simulink model "Sampling_switch_uncertainty"  (R2021b)
settings: Solver=VariableStepAuto  StartTime=0.0  StopTime=10.0  RelTol=1e-3
values from neighbouring files (symbols this model uses):
  bits_number = 13    [launch_pipeline_switch.m]
  cst = 2*pi*fin/1000    [launch_pipeline_switch.m]
  fin = antismear(fin_pre,fs,nfft)    [launch_pipeline_switch.m]
  ts = 1/fs    (= 1)    [launch_pipeline_switch.m]
(part 1 of 2)
settings Model: Creator=86151  LastModifiedBy=86151

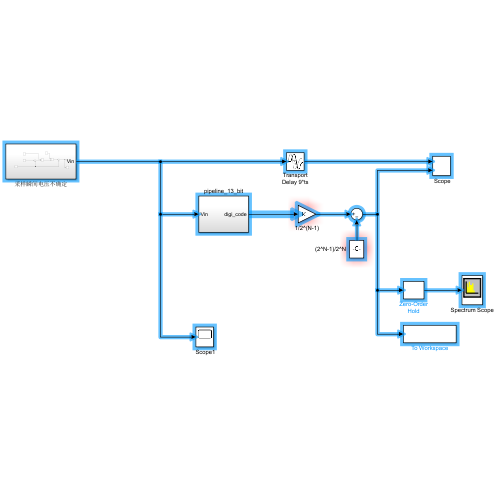
[thumbnail: Simulink's stored preview of the top-level diagram]
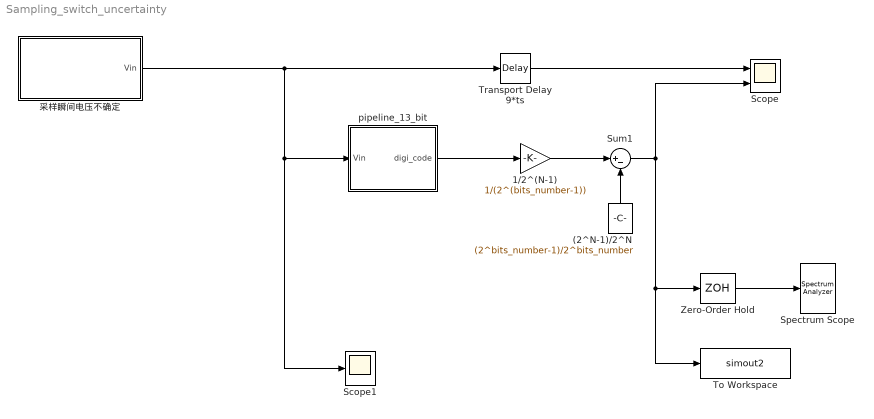
== system Sampling_switch_uncertainty ==
  " Scope" : Scope  NumInputPorts=2
  " Scope1" : Scope
  (2^N-1)/2^N : Constant  Value=(2^bits_number-1)/2^bits_number
  1/2^(N-1) : Gain  Gain=1/(2^(bits_number-1))
  Spectrum Scope : SpectrumAnalyzer
  Sum1 : Sum  Inputs=|+-
  To Workspace : ToWorkspace  VariableName=simout2  SampleTime=-1
  Transport Delay 9*ts : TransportDelay  DelayTime=9
  Zero-Order Hold : ZeroOrderHold
  pipeline_13_bit : Subsystem
  采样瞬间电压不确定 : Subsystem
  wires:
  采样瞬间电压不确定/1(Vin) -> " Scope1"/1, pipeline_13_bit/1(Vin), Transport Delay 9*ts/1
  Transport Delay 9*ts/1 -> " Scope"/1
  Zero-Order Hold/1 -> Spectrum Scope/1
  Sum1/1 -> " Scope"/2, To Workspace/1, Zero-Order Hold/1
  (2^N-1)/2^N/1 -> Sum1/2
  1/2^(N-1)/1 -> Sum1/1
  pipeline_13_bit/1(digi_code) -> 1/2^(N-1)/1

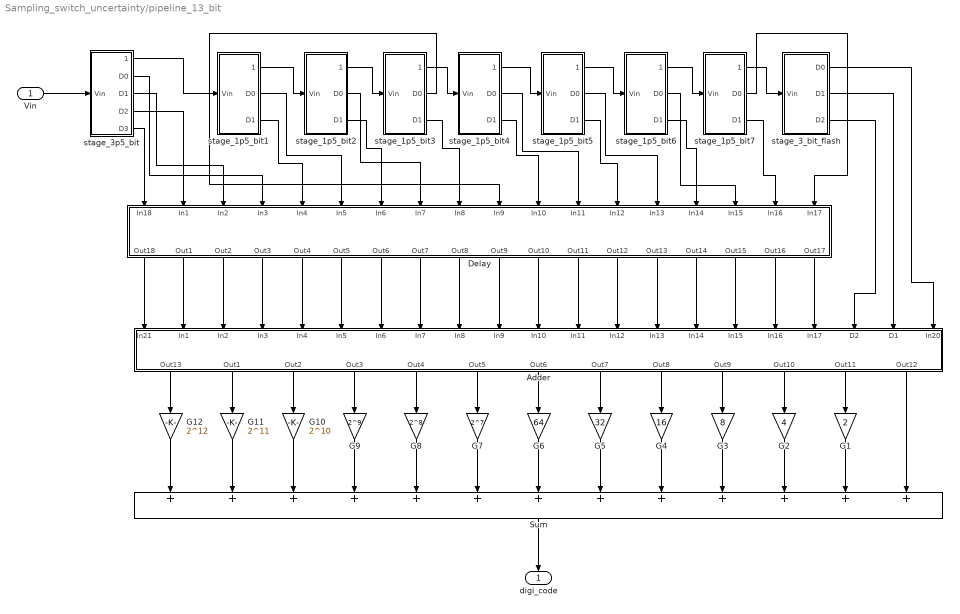
== system Sampling_switch_uncertainty/pipeline_13_bit ==
  Vin : Inport
  Adder : Subsystem
  Delay : Subsystem
  G1 : Gain  Gain=2
  G10 : Gain  Gain=2^10
  G11 : Gain  Gain=2^11
  G12 : Gain  Gain=2^12
  G2 : Gain  Gain=4
  G3 : Gain  Gain=8
  G4 : Gain  Gain=16
  G5 : Gain  Gain=32
  G6 : Gain  Gain=64
  G7 : Gain  Gain=2^7
  G8 : Gain  Gain=2^8
  G9 : Gain  Gain=2^9
  Sum : Sum  Inputs=+++++++++++++
  stage_1p5_bit1 : Subsystem
  stage_1p5_bit2 : Subsystem
  stage_1p5_bit3 : Subsystem
  stage_1p5_bit4 : Subsystem
  stage_1p5_bit5 : Subsystem
  stage_1p5_bit6 : Subsystem
  stage_1p5_bit7 : Subsystem
  stage_3_bit_flash : Subsystem
  stage_3p5_bit : Subsystem
  digi_code : Outport
  wires:
  G1/1 -> Sum/12
  stage_3p5_bit/4(D2) -> Delay/2(In1)
  stage_3p5_bit/3(D1) -> Delay/3(In2)
  stage_3p5_bit/2(D0) -> Delay/4(In3)
  stage_1p5_bit1/3(D1) -> Delay/5(In4)
  stage_1p5_bit1/2(D0) -> Delay/6(In5)
  stage_1p5_bit2/3(D1) -> Delay/7(In6)
  stage_1p5_bit2/2(D0) -> Delay/8(In7)
  G2/1 -> Sum/11
  G3/1 -> Sum/10
  G4/1 -> Sum/9
  G5/1 -> Sum/8
  G6/1 -> Sum/7
  G7/1 -> Sum/6
  G8/1 -> Sum/5
  G9/1 -> Sum/4
  G10/1 -> Sum/3
  G11/1 -> Sum/2
  stage_3_bit_flash/1(D0) -> Adder/21(In20)
  Adder/2(Out1) -> G11/1
  Adder/3(Out2) -> G10/1
  Adder/4(Out3) -> G9/1
  Adder/5(Out4) -> G8/1
  Adder/6(Out5) -> G7/1
  Adder/13(Out12) -> Sum/13
  Adder/12(Out11) -> G1/1
  Adder/11(Out10) -> G2/1
  Adder/10(Out9) -> G3/1
  Adder/9(Out8) -> G4/1
  Adder/8(Out7) -> G5/1
  Adder/7(Out6) -> G6/1
  stage_1p5_bit1/1(Residue) -> stage_1p5_bit2/1(Vin)
  stage_1p5_bit2/1(Residue) -> stage_1p5_bit3/1(Vin)
  stage_1p5_bit3/1(Residue) -> stage_1p5_bit4/1(Vin)
  stage_1p5_bit4/1(Residue) -> stage_1p5_bit5/1(Vin)
  stage_3p5_bit/1(Residue) -> stage_1p5_bit1/1(Vin)
  stage_1p5_bit5/1(Residue) -> stage_1p5_bit6/1(Vin)
  stage_1p5_bit7/1(Residue) -> stage_3_bit_flash/1(Vin)
  stage_1p5_bit6/1(Residue) -> stage_1p5_bit7/1(Vin)
  Vin/1 -> stage_3p5_bit/1(Vin)
  Sum/1 -> digi_code/1
  stage_1p5_bit3/3(D1) -> Delay/9(In8)
  stage_1p5_bit3/2(D0) -> Delay/10(In9)
  stage_1p5_bit4/3(D1) -> Delay/11(In10)
  stage_1p5_bit4/2(D0) -> Delay/12(In11)
  stage_1p5_bit7/2(D0) -> Delay/18(In17)
  stage_1p5_bit7/3(D1) -> Delay/17(In16)
  stage_1p5_bit6/2(D0) -> Delay/16(In15)
  stage_1p5_bit6/3(D1) -> Delay/15(In14)
  stage_1p5_bit5/2(D0) -> Delay/14(In13)
  stage_1p5_bit5/3(D1) -> Delay/13(In12)
  Delay/2(Out1) -> Adder/2(In1)
  Delay/3(Out2) -> Adder/3(In2)
  Delay/4(Out3) -> Adder/4(In3)
  Delay/5(Out4) -> Adder/5(In4)
  Delay/6(Out5) -> Adder/6(In5)
  Delay/7(Out6) -> Adder/7(In6)
  Delay/8(Out7) -> Adder/8(In7)
  Delay/9(Out8) -> Adder/9(In8)
  Delay/10(Out9) -> Adder/10(In9)
  Delay/11(Out10) -> Adder/11(In10)
  Delay/13(Out12) -> Adder/13(In12)
  Delay/14(Out13) -> Adder/14(In13)
  Delay/15(Out14) -> Adder/15(In14)
  Delay/16(Out15) -> Adder/16(In15)
  Delay/17(Out16) -> Adder/17(In16)
  Delay/18(Out17) -> Adder/18(In17)
  Delay/12(Out11) -> Adder/12(In11)
  stage_3p5_bit/5(D3) -> Delay/1(In18)
  Delay/1(Out18) -> Adder/1(In21)
  stage_3_bit_flash/2(D1) -> Adder/20(D1)
  stage_3_bit_flash/3(D2) -> Adder/19(D2)
  Adder/1(Out13) -> G12/1
  G12/1 -> Sum/1

== system Sampling_switch_uncertainty/采样瞬间电压不确定 ==
  " Scope1" : Scope
  Constant : Constant
  Constant1 : Constant  Value=cst
  Product : Product
  Product1 : Product
  Sine Wave w fin = 0.1 Hz (set in launch.m)1 : Sin  Bias=pi/2  Frequency=2*pi*fin  SampleTime=0
  Sine Wave w fin = 0.1 Hz (set in launch.m)2 : Sin  Frequency=2*pi*fin  SampleTime=0
  Sum : Sum  Inputs=|+-
  Sum2 : Sum  Inputs=|++
  Vin : Outport
  wires:
  Sine Wave w fin = 0.1 Hz (set in launch.m)2/1 -> Sum2/2, Sum/2
  Constant/1 -> Sum/1
  Constant1/1 -> Product1/1
  Sum/1 -> Product/2
  Product/1 -> Product1/2
  Product1/1 -> Sum2/1
  Sine Wave w fin = 0.1 Hz (set in launch.m)1/1 -> Product/1
  Sum2/1 -> " Scope1"/1, Vin/1

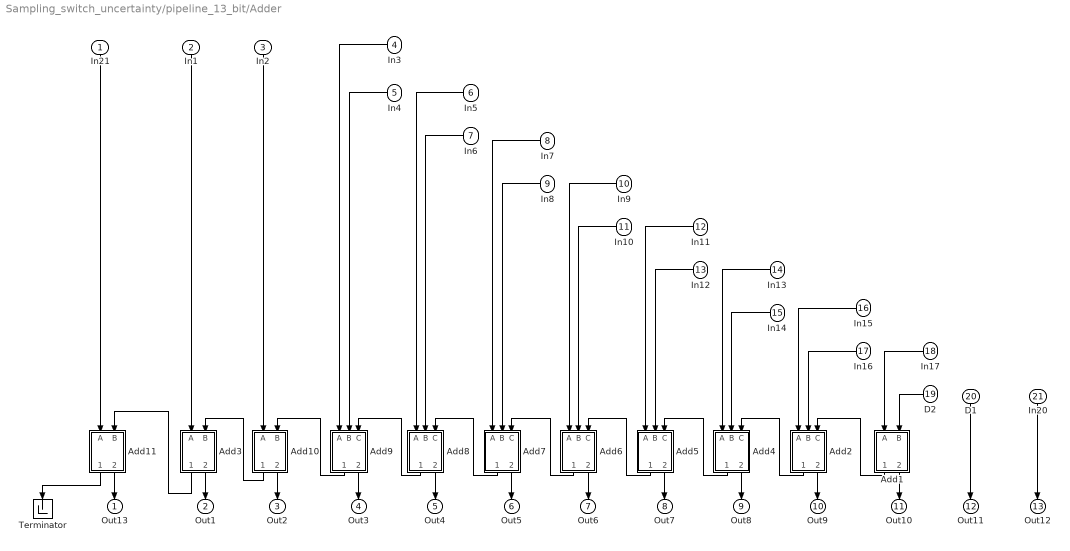
== system Sampling_switch_uncertainty/pipeline_13_bit/Adder ==
  In21 : Inport
  In1 : Inport  Port=2
  In2 : Inport  Port=3
  In3 : Inport  Port=4
  In4 : Inport  Port=5
  In5 : Inport  Port=6
  In6 : Inport  Port=7
  In7 : Inport  Port=8
  In8 : Inport  Port=9
  In9 : Inport  Port=10
  In10 : Inport  Port=11
  In11 : Inport  Port=12
  In12 : Inport  Port=13
  In13 : Inport  Port=14
  In14 : Inport  Port=15
  In15 : Inport  Port=16
  In16 : Inport  Port=17
  In17 : Inport  Port=18
  D2 : Inport  Port=19
  D1 : Inport  Port=20
  In20 : Inport  Port=21
  Add1 : Subsystem
  Add10 : Subsystem
  Add11 : Subsystem
  Add2 : Subsystem
  Add3 : Subsystem
  Add4 : Subsystem
  Add5 : Subsystem
  Add6 : Subsystem
  Add7 : Subsystem
  Add8 : Subsystem
  Add9 : Subsystem
  Terminator : Terminator
  Out13 : Outport
  Out1 : Outport  Port=2
  Out2 : Outport  Port=3
  Out3 : Outport  Port=4
  Out4 : Outport  Port=5
  Out5 : Outport  Port=6
  Out6 : Outport  Port=7
  Out7 : Outport  Port=8
  Out8 : Outport  Port=9
  Out9 : Outport  Port=10
  Out10 : Outport  Port=11
  Out11 : Outport  Port=12
  Out12 : Outport  Port=13
  wires:
  In20/1 -> Out12/1
  D1/1 -> Out11/1
  D2/1 -> Add1/2(B)
  In17/1 -> Add1/1(A)
  Add1/2(Sum) -> Out10/1
  Add1/1(Carry) -> Add2/3(C)
  Add2/2(Sum) -> Out9/1
  In14/1 -> Add4/2(B)
  In13/1 -> Add4/1(A)
  Add5/2(Sum) -> Out7/1
  Add4/1(Carry) -> Add5/3(C)
  In12/1 -> Add5/2(B)
  In11/1 -> Add5/1(A)
  Add6/2(Sum) -> Out6/1
  Add5/1(Carry) -> Add6/3(C)
  In10/1 -> Add6/2(B)
  In9/1 -> Add6/1(A)
  Add7/2(Sum) -> Out5/1
  Add6/1(Carry) -> Add7/3(C)
  In8/1 -> Add7/2(B)
  In7/1 -> Add7/1(A)
  Add8/2(Sum) -> Out4/1
  Add7/1(Carry) -> Add8/3(C)
  In6/1 -> Add8/2(B)
  In5/1 -> Add8/1(A)
  Add8/1(Carry) -> Add9/3(C)
  Add9/2(Sum) -> Out3/1
  In4/1 -> Add9/2(B)
  In3/1 -> Add9/1(A)
  Add10/2(Sum) -> Out2/1
  Add9/1(Carry) -> Add10/2(B)
  In2/1 -> Add10/1(A)
  In16/1 -> Add2/2(B)
  In15/1 -> Add2/1(A)
  Add2/1(Carry) -> Add4/3(C)
  Add4/2(Sum) -> Out8/1
  Add10/1(Carry) -> Add3/2(B)
  Add3/2(Sum) -> Out1/1
  In1/1 -> Add3/1(A)
  In21/1 -> Add11/1(A)
  Add11/2(Sum) -> Out13/1
  Add3/1(Carry) -> Add11/2(B)
  Add11/1(Carry) -> Terminator/1

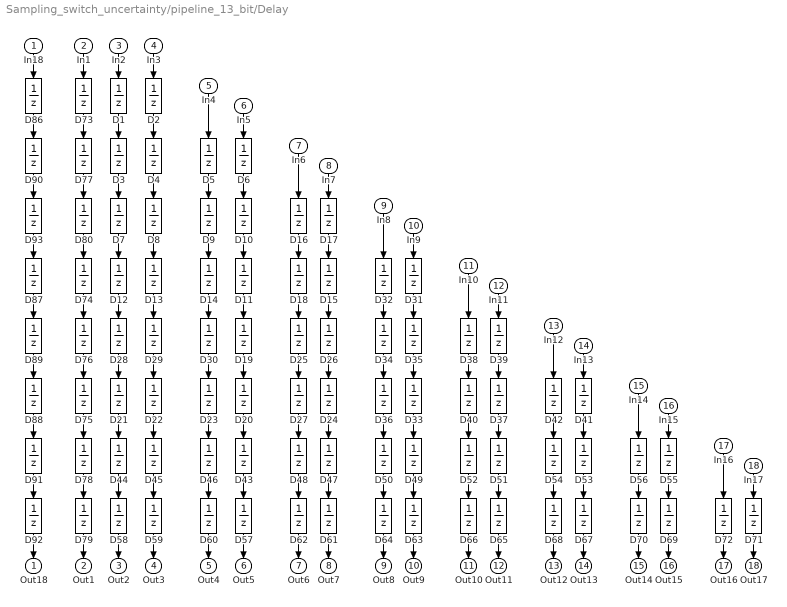
== system Sampling_switch_uncertainty/pipeline_13_bit/Delay ==
  In18 : Inport
  In1 : Inport  Port=2
  In2 : Inport  Port=3
  In3 : Inport  Port=4
  In4 : Inport  Port=5
  In5 : Inport  Port=6
  In6 : Inport  Port=7
  In7 : Inport  Port=8
  In8 : Inport  Port=9
  In9 : Inport  Port=10
  In10 : Inport  Port=11
  In11 : Inport  Port=12
  In12 : Inport  Port=13
  In13 : Inport  Port=14
  In14 : Inport  Port=15
  In15 : Inport  Port=16
  In16 : Inport  Port=17
  In17 : Inport  Port=18
  D{1..80,86..93} (88 alike) : UnitDelay  SampleTime=-1  HasFrameUpgradeWarning=on
  Out18 : Outport
  Out1 : Outport  Port=2
  Out2 : Outport  Port=3
  Out3 : Outport  Port=4
  Out4 : Outport  Port=5
  Out5 : Outport  Port=6
  Out6 : Outport  Port=7
  Out7 : Outport  Port=8
  Out8 : Outport  Port=9
  Out9 : Outport  Port=10
  Out10 : Outport  Port=11
  Out11 : Outport  Port=12
  Out12 : Outport  Port=13
  Out13 : Outport  Port=14
  Out14 : Outport  Port=15
  Out15 : Outport  Port=16
  Out16 : Outport  Port=17
  Out17 : Outport  Port=18
  wires:
  D2/1 -> D4/1
  D1/1 -> D3/1
  In2/1 -> D1/1
  In3/1 -> D2/1
  In5/1 -> D6/1
  In4/1 -> D5/1
  D4/1 -> D8/1
  D3/1 -> D7/1
  D6/1 -> D10/1
  D5/1 -> D9/1
  D8/1 -> D13/1
  D7/1 -> D12/1
  D10/1 -> D11/1
  D9/1 -> D14/1
  In7/1 -> D17/1
  In6/1 -> D16/1
  D17/1 -> D15/1
  D16/1 -> D18/1
  D15/1 -> D26/1
  D18/1 -> D25/1
  D13/1 -> D29/1
  D12/1 -> D28/1
  D11/1 -> D19/1
  D14/1 -> D30/1
  D29/1 -> D22/1
  D28/1 -> D21/1
  D19/1 -> D20/1
  D30/1 -> D23/1
  D26/1 -> D24/1
  D25/1 -> D27/1
  D24/1 -> D47/1
  D27/1 -> D48/1
  D31/1 -> D35/1
  D32/1 -> D34/1
  D35/1 -> D33/1
  D34/1 -> D36/1
  D33/1 -> D49/1
  D36/1 -> D50/1
  D39/1 -> D37/1
  D38/1 -> D40/1
  D37/1 -> D51/1
  D40/1 -> D52/1
  D41/1 -> D53/1
  D42/1 -> D54/1
  D47/1 -> D61/1
  D49/1 -> D63/1
  D50/1 -> D64/1
  D51/1 -> D65/1
  D52/1 -> D66/1
  D53/1 -> D67/1
  D54/1 -> D68/1
  D21/1 -> D44/1
  D22/1 -> D45/1
  D23/1 -> D46/1
  D20/1 -> D43/1
  In15/1 -> D55/1
  In14/1 -> D56/1
  D55/1 -> D69/1
  D56/1 -> D70/1
  D61/1 -> Out7/1
  D62/1 -> Out6/1
  D63/1 -> Out9/1
  D64/1 -> Out8/1
  D65/1 -> Out11/1
  D66/1 -> Out10/1
  D67/1 -> Out13/1
  D68/1 -> Out12/1
  D44/1 -> D58/1
  D45/1 -> D59/1
  D46/1 -> D60/1
  D43/1 -> D57/1
  D69/1 -> Out15/1
  D70/1 -> Out14/1
  D48/1 -> D62/1
  D71/1 -> Out17/1
  D72/1 -> Out16/1
  D73/1 -> D77/1
  D77/1 -> D80/1
  D80/1 -> D74/1
  D74/1 -> D76/1
  D76/1 -> D75/1
  D75/1 -> D78/1
  D78/1 -> D79/1
  In1/1 -> D73/1
  In8/1 -> D32/1
  In17/1 -> D71/1
  In16/1 -> D72/1
  In13/1 -> D41/1
  In12/1 -> D42/1
  In11/1 -> D39/1
  In10/1 -> D38/1
  In9/1 -> D31/1
  D79/1 -> Out1/1
  D58/1 -> Out2/1
  D59/1 -> Out3/1
  D60/1 -> Out4/1
  D57/1 -> Out5/1
  D90/1 -> D93/1
  In18/1 -> D86/1
  D88/1 -> D91/1
  D89/1 -> D88/1
  D91/1 -> D92/1
  D92/1 -> Out18/1
  D87/1 -> D89/1
  D86/1 -> D90/1
  D93/1 -> D87/1

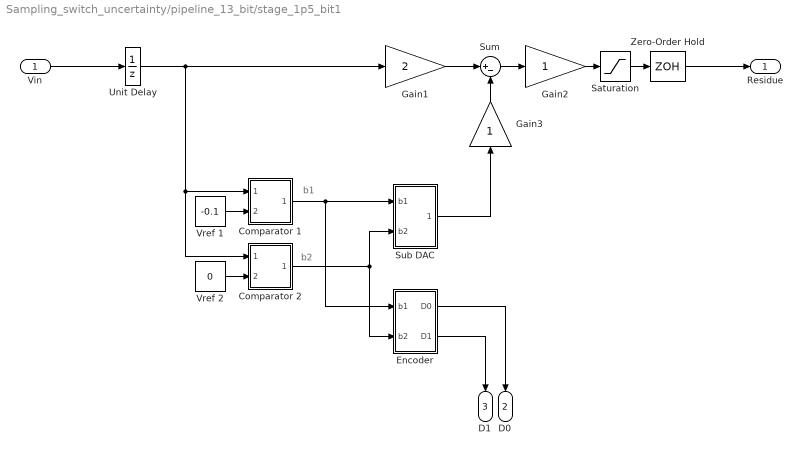
== system Sampling_switch_uncertainty/pipeline_13_bit/stage_1p5_bit1 ==
  note: b2
  note: b1
  Vin : Inport
  Comparator 1 : Subsystem
  Comparator 2 : Subsystem
  Encoder : Subsystem
  Gain1 : Gain  Gain=2
  Gain2 : Gain
  Gain3 : Gain
  Saturation : Saturate  UpperLimit=1  LowerLimit=-1
  Sub DAC : Subsystem
  Sum : Sum  Inputs=|+-
  Unit Delay : UnitDelay  SampleTime=-1  HasFrameUpgradeWarning=on
  Vref 1 : Constant  Value=-0.1
  Vref 2 : Constant  Value=0
  Zero-Order Hold : ZeroOrderHold  SampleTime=ts
  Residue : Outport
  D0 : Outport  Port=2
  D1 : Outport  Port=3
  wires:
  Vref 1/1 -> Comparator 1/2(Vref)
  Gain1/1 -> Sum/1
  Gain3/1 -> Sum/2
  Sum/1 -> Gain2/1
  Saturation/1 -> Zero-Order Hold/1
  Zero-Order Hold/1 -> Residue/1
  Gain2/1 -> Saturation/1
  Vref 2/1 -> Comparator 2/2(Vref)
  Comparator 2/1(Out) -> Sub DAC/2(b2), Encoder/2(b2)
  Vin/1 -> Unit Delay/1
  Comparator 1/1(Out) -> Encoder/1(b1), Sub DAC/1(b1)
  Unit Delay/1 -> Comparator 1/1(Vin), Comparator 2/1(Vin), Gain1/1
  Sub DAC/1(Vdac) -> Gain3/1
  Encoder/1(D0) -> D0/1
  Encoder/2(D1) -> D1/1

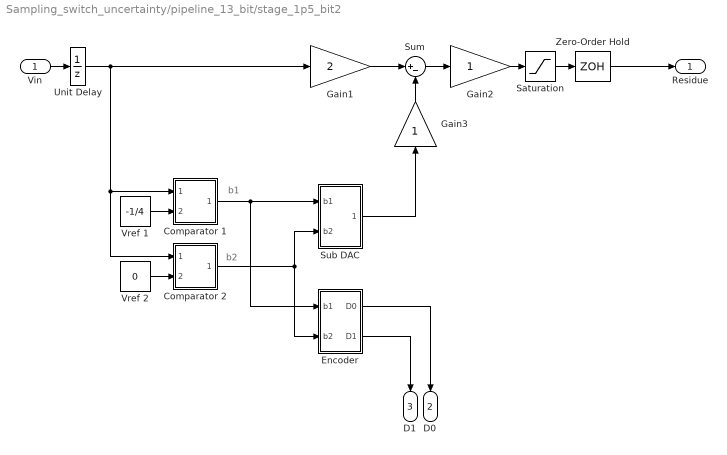
== system Sampling_switch_uncertainty/pipeline_13_bit/stage_1p5_bit2 ==
  note: b2
  note: b1
  Vin : Inport
  Comparator 1 : Subsystem
  Comparator 2 : Subsystem
  Encoder : Subsystem
  Gain1 : Gain  Gain=2
  Gain2 : Gain
  Gain3 : Gain
  Saturation : Saturate  UpperLimit=1  LowerLimit=-1
  Sub DAC : Subsystem
  Sum : Sum  Inputs=|+-
  Unit Delay : UnitDelay  SampleTime=-1  HasFrameUpgradeWarning=on
  Vref 1 : Constant  Value=-1/4
  Vref 2 : Constant  Value=0
  Zero-Order Hold : ZeroOrderHold  SampleTime=ts
  Residue : Outport
  D0 : Outport  Port=2
  D1 : Outport  Port=3
  wires:
  Vref 1/1 -> Comparator 1/2(Vref)
  Gain1/1 -> Sum/1
  Gain3/1 -> Sum/2
  Sum/1 -> Gain2/1
  Saturation/1 -> Zero-Order Hold/1
  Zero-Order Hold/1 -> Residue/1
  Gain2/1 -> Saturation/1
  Vref 2/1 -> Comparator 2/2(Vref)
  Comparator 2/1(Out) -> Sub DAC/2(b2), Encoder/2(b2)
  Vin/1 -> Unit Delay/1
  Comparator 1/1(Out) -> Encoder/1(b1), Sub DAC/1(b1)
  Unit Delay/1 -> Comparator 1/1(Vin), Comparator 2/1(Vin), Gain1/1
  Sub DAC/1(Vdac) -> Gain3/1
  Encoder/1(D0) -> D0/1
  Encoder/2(D1) -> D1/1

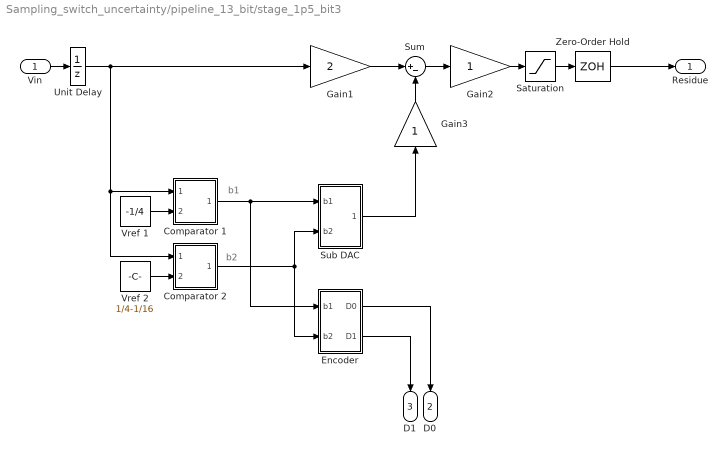
== system Sampling_switch_uncertainty/pipeline_13_bit/stage_1p5_bit3 ==
  note: b2
  note: b1
  Vin : Inport
  Comparator 1 : Subsystem
  Comparator 2 : Subsystem
  Encoder : Subsystem
  Gain1 : Gain  Gain=2
  Gain2 : Gain
  Gain3 : Gain
  Saturation : Saturate  UpperLimit=1  LowerLimit=-1
  Sub DAC : Subsystem
  Sum : Sum  Inputs=|+-
  Unit Delay : UnitDelay  SampleTime=-1  HasFrameUpgradeWarning=on
  Vref 1 : Constant  Value=-1/4
  Vref 2 : Constant  Value=1/4-1/16
  Zero-Order Hold : ZeroOrderHold  SampleTime=ts
  Residue : Outport
  D0 : Outport  Port=2
  D1 : Outport  Port=3
  wires:
  Vref 1/1 -> Comparator 1/2(Vref)
  Gain1/1 -> Sum/1
  Gain3/1 -> Sum/2
  Sum/1 -> Gain2/1
  Saturation/1 -> Zero-Order Hold/1
  Zero-Order Hold/1 -> Residue/1
  Gain2/1 -> Saturation/1
  Vref 2/1 -> Comparator 2/2(Vref)
  Comparator 2/1(Out) -> Sub DAC/2(b2), Encoder/2(b2)
  Vin/1 -> Unit Delay/1
  Comparator 1/1(Out) -> Encoder/1(b1), Sub DAC/1(b1)
  Unit Delay/1 -> Comparator 1/1(Vin), Comparator 2/1(Vin), Gain1/1
  Sub DAC/1(Vdac) -> Gain3/1
  Encoder/1(D0) -> D0/1
  Encoder/2(D1) -> D1/1

== system Sampling_switch_uncertainty/pipeline_13_bit/stage_1p5_bit4 ==
  note: b2
  note: b1
  Vin : Inport
  Comparator 1 : Subsystem
  Comparator 2 : Subsystem
  Encoder : Subsystem
  Gain1 : Gain  Gain=2
  Gain2 : Gain
  Gain3 : Gain
  Saturation : Saturate  UpperLimit=1  LowerLimit=-1
  Sub DAC : Subsystem
  Sum : Sum  Inputs=|+-
  Unit Delay : UnitDelay  SampleTime=-1  HasFrameUpgradeWarning=on
  Vref 1 : Constant  Value=-1/4
  Vref 2 : Constant  Value=1/4-1/16
  Zero-Order Hold : ZeroOrderHold  SampleTime=ts
  Residue : Outport
  D0 : Outport  Port=2
  D1 : Outport  Port=3
  wires:
  Vref 1/1 -> Comparator 1/2(Vref)
  Gain1/1 -> Sum/1
  Gain3/1 -> Sum/2
  Sum/1 -> Gain2/1
  Saturation/1 -> Zero-Order Hold/1
  Zero-Order Hold/1 -> Residue/1
  Gain2/1 -> Saturation/1
  Vref 2/1 -> Comparator 2/2(Vref)
  Comparator 2/1(Out) -> Sub DAC/2(b2), Encoder/2(b2)
  Vin/1 -> Unit Delay/1
  Comparator 1/1(Out) -> Encoder/1(b1), Sub DAC/1(b1)
  Unit Delay/1 -> Comparator 1/1(Vin), Comparator 2/1(Vin), Gain1/1
  Sub DAC/1(Vdac) -> Gain3/1
  Encoder/1(D0) -> D0/1
  Encoder/2(D1) -> D1/1

== system Sampling_switch_uncertainty/pipeline_13_bit/stage_1p5_bit5 ==
  note: b2
  note: b1
  Vin : Inport
  Comparator 1 : Subsystem
  Comparator 2 : Subsystem
  Encoder : Subsystem
  Gain1 : Gain  Gain=2
  Gain2 : Gain
  Gain3 : Gain
  Saturation : Saturate  UpperLimit=1  LowerLimit=-1
  Sub DAC : Subsystem
  Sum : Sum  Inputs=|+-
  Unit Delay : UnitDelay  SampleTime=-1  HasFrameUpgradeWarning=on
  Vref 1 : Constant  Value=-1/4
  Vref 2 : Constant  Value=1/4-1/16
  Zero-Order Hold : ZeroOrderHold  SampleTime=ts
  Residue : Outport
  D0 : Outport  Port=2
  D1 : Outport  Port=3
  wires:
  Vref 1/1 -> Comparator 1/2(Vref)
  Gain1/1 -> Sum/1
  Gain3/1 -> Sum/2
  Sum/1 -> Gain2/1
  Saturation/1 -> Zero-Order Hold/1
  Zero-Order Hold/1 -> Residue/1
  Gain2/1 -> Saturation/1
  Vref 2/1 -> Comparator 2/2(Vref)
  Comparator 2/1(Out) -> Sub DAC/2(b2), Encoder/2(b2)
  Vin/1 -> Unit Delay/1
  Comparator 1/1(Out) -> Encoder/1(b1), Sub DAC/1(b1)
  Unit Delay/1 -> Comparator 1/1(Vin), Comparator 2/1(Vin), Gain1/1
  Sub DAC/1(Vdac) -> Gain3/1
  Encoder/1(D0) -> D0/1
  Encoder/2(D1) -> D1/1

== system Sampling_switch_uncertainty/pipeline_13_bit/stage_1p5_bit6 ==
  note: b2
  note: b1
  Vin : Inport
  Comparator 1 : Subsystem
  Comparator 2 : Subsystem
  Encoder : Subsystem
  Gain1 : Gain  Gain=2
  Gain2 : Gain
  Gain3 : Gain
  Saturation : Saturate  UpperLimit=1  LowerLimit=-1
  Sub DAC : Subsystem
  Sum : Sum  Inputs=|+-
  Unit Delay : UnitDelay  SampleTime=-1  HasFrameUpgradeWarning=on
  Vref 1 : Constant  Value=-1/4
  Vref 2 : Constant  Value=1/4
  Zero-Order Hold : ZeroOrderHold  SampleTime=ts
  Residue : Outport
  D0 : Outport  Port=2
  D1 : Outport  Port=3
  wires:
  Vref 1/1 -> Comparator 1/2(Vref)
  Gain1/1 -> Sum/1
  Gain3/1 -> Sum/2
  Sum/1 -> Gain2/1
  Saturation/1 -> Zero-Order Hold/1
  Zero-Order Hold/1 -> Residue/1
  Gain2/1 -> Saturation/1
  Vref 2/1 -> Comparator 2/2(Vref)
  Comparator 2/1(Out) -> Sub DAC/2(b2), Encoder/2(b2)
  Vin/1 -> Unit Delay/1
  Comparator 1/1(Out) -> Encoder/1(b1), Sub DAC/1(b1)
  Unit Delay/1 -> Comparator 1/1(Vin), Comparator 2/1(Vin), Gain1/1
  Sub DAC/1(Vdac) -> Gain3/1
  Encoder/1(D0) -> D0/1
  Encoder/2(D1) -> D1/1

== system Sampling_switch_uncertainty/pipeline_13_bit/stage_1p5_bit7 ==
  note: b2
  note: b1
  Vin : Inport
  Comparator 1 : Subsystem
  Comparator 2 : Subsystem
  Encoder : Subsystem
  Gain1 : Gain  Gain=2
  Gain2 : Gain
  Gain3 : Gain
  Saturation : Saturate  UpperLimit=1  LowerLimit=-1
  Sub DAC : Subsystem
  Sum : Sum  Inputs=|+-
  Unit Delay : UnitDelay  SampleTime=-1  HasFrameUpgradeWarning=on
  Vref 1 : Constant  Value=-1/4
  Vref 2 : Constant  Value=0
  Zero-Order Hold : ZeroOrderHold  SampleTime=ts
  Residue : Outport
  D0 : Outport  Port=2
  D1 : Outport  Port=3
  wires:
  Vref 1/1 -> Comparator 1/2(Vref)
  Gain1/1 -> Sum/1
  Gain3/1 -> Sum/2
  Sum/1 -> Gain2/1
  Saturation/1 -> Zero-Order Hold/1
  Zero-Order Hold/1 -> Residue/1
  Gain2/1 -> Saturation/1
  Vref 2/1 -> Comparator 2/2(Vref)
  Comparator 2/1(Out) -> Sub DAC/2(b2), Encoder/2(b2)
  Vin/1 -> Unit Delay/1
  Comparator 1/1(Out) -> Encoder/1(b1), Sub DAC/1(b1)
  Unit Delay/1 -> Comparator 1/1(Vin), Comparator 2/1(Vin), Gain1/1
  Sub DAC/1(Vdac) -> Gain3/1
  Encoder/1(D0) -> D0/1
  Encoder/2(D1) -> D1/1

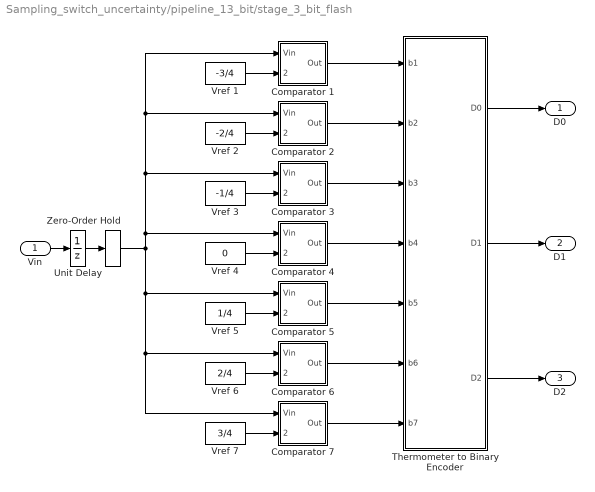
== system Sampling_switch_uncertainty/pipeline_13_bit/stage_3_bit_flash ==
  Vin : Inport
  Comparator 1 : Subsystem
  Comparator 2 : Subsystem
  Comparator 3 : Subsystem
  Comparator 4 : Subsystem
  Comparator 5 : Subsystem
  Comparator 6 : Subsystem
  Comparator 7 : Subsystem
  Thermometer to Binary Encoder : Subsystem
  Unit Delay : UnitDelay  SampleTime=-1  HasFrameUpgradeWarning=on
  Vref 1 : Constant  Value=-3/4
  Vref 2 : Constant  Value=-2/4
  Vref 3 : Constant  Value=-1/4
  Vref 4 : Constant  Value=0
  Vref 5 : Constant  Value=1/4
  Vref 6 : Constant  Value=2/4
  Vref 7 : Constant  Value=3/4
  Zero-Order Hold : ZeroOrderHold  SampleTime=ts
  D0 : Outport
  D1 : Outport  Port=2
  D2 : Outport  Port=3
  wires:
  Vin/1 -> Unit Delay/1
  Vref 1/1 -> Comparator 1/2(Vref)
  Thermometer to Binary Encoder/1(D0) -> D0/1
  Thermometer to Binary Encoder/2(D1) -> D1/1
  Thermometer to Binary Encoder/3(D2) -> D2/1
  Comparator 1/1(Out) -> Thermometer to Binary Encoder/1(b1)
  Vref 2/1 -> Comparator 2/2(Vref)
  Comparator 2/1(Out) -> Thermometer to Binary Encoder/2(b2)
  Vref 3/1 -> Comparator 3/2(Vref)
  Comparator 3/1(Out) -> Thermometer to Binary Encoder/3(b3)
  Vref 4/1 -> Comparator 4/2(Vref)
  Comparator 4/1(Out) -> Thermometer to Binary Encoder/4(b4)
  Vref 5/1 -> Comparator 5/2(Vref)
  Comparator 5/1(Out) -> Thermometer to Binary Encoder/5(b5)
  Vref 6/1 -> Comparator 6/2(Vref)
  Comparator 6/1(Out) -> Thermometer to Binary Encoder/6(b6)
  Vref 7/1 -> Comparator 7/2(Vref)
  Comparator 7/1(Out) -> Thermometer to Binary Encoder/7(b7)
  Zero-Order Hold/1 -> Comparator 1/1(Vin), Comparator 2/1(Vin), Comparator 3/1(Vin), Comparator 4/1(Vin), Comparator 5/1(Vin), Comparator 6/1(Vin), Comparator 7/1(Vin)
  Unit Delay/1 -> Zero-Order Hold/1

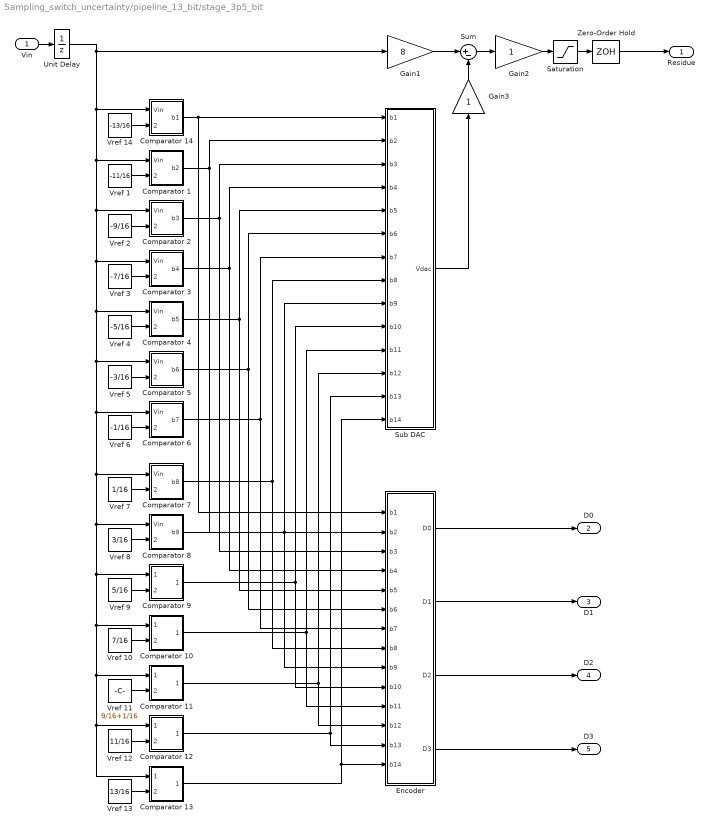
== system Sampling_switch_uncertainty/pipeline_13_bit/stage_3p5_bit ==
  Vin : Inport
  Comparator 1 : Subsystem
  Comparator 10 : Subsystem
  Comparator 11 : Subsystem
  Comparator 12 : Subsystem
  Comparator 13 : Subsystem
  Comparator 14 : Subsystem
  Comparator 2 : Subsystem
  Comparator 3 : Subsystem
  Comparator 4 : Subsystem
  Comparator 5 : Subsystem
  Comparator 6 : Subsystem
  Comparator 7 : Subsystem
  Comparator 8 : Subsystem
  Comparator 9 : Subsystem
  Encoder : Subsystem
  Gain1 : Gain  Gain=8
  Gain2 : Gain
  Gain3 : Gain
  Saturation : Saturate  UpperLimit=1  LowerLimit=-1
  Sub DAC : Subsystem
  Sum : Sum  Inputs=|+-
  Unit Delay : UnitDelay  SampleTime=-1  HasFrameUpgradeWarning=on
  Vref 1 : Constant  Value=-11/16
  Vref 10 : Constant  Value=7/16
  Vref 11 : Constant  Value=9/16+1/16
  Vref 12 : Constant  Value=11/16
  Vref 13 : Constant  Value=13/16
  Vref 14 : Constant  Value=-13/16
  Vref 2 : Constant  Value=-9/16
  Vref 3 : Constant  Value=-7/16
  Vref 4 : Constant  Value=-5/16
  Vref 5 : Constant  Value=-3/16
  Vref 6 : Constant  Value=-1/16
  Vref 7 : Constant  Value=1/16
  Vref 8 : Constant  Value=3/16
  Vref 9 : Constant  Value=5/16
  Zero-Order Hold : ZeroOrderHold  SampleTime=ts
  Residue : Outport
  D0 : Outport  Port=2
  D1 : Outport  Port=3
  D2 : Outport  Port=4
  D3 : Outport  Port=5
  wires:
  Vref 1/1 -> Comparator 1/2(Vref)
  Sub DAC/1(Vdac) -> Gain3/1
  Gain1/1 -> Sum/1
  Gain3/1 -> Sum/2
  Sum/1 -> Gain2/1
  Saturation/1 -> Zero-Order Hold/1
  Zero-Order Hold/1 -> Residue/1
  Gain2/1 -> Saturation/1
  Vref 2/1 -> Comparator 2/2(Vref)
  Vin/1 -> Unit Delay/1
  Vref 3/1 -> Comparator 3/2(Vref)
  Vref 4/1 -> Comparator 4/2(Vref)
  Vref 5/1 -> Comparator 5/2(Vref)
  Vref 6/1 -> Comparator 6/2(Vref)
  Encoder/1(D0) -> D0/1
  Encoder/3(D2) -> D2/1
  Encoder/2(D1) -> D1/1
  Vref 10/1 -> Comparator 10/2(Vref)
  Vref 12/1 -> Comparator 12/2(Vref)
  Vref 11/1 -> Comparator 11/2(Vref)
  Vref 8/1 -> Comparator 8/2(Vref)
  Vref 7/1 -> Comparator 7/2(Vref)
  Vref 9/1 -> Comparator 9/2(Vref)
  Vref 13/1 -> Comparator 13/2(Vref)
  Unit Delay/1 -> Comparator 14/1(Vin), Comparator 1/1(Vin), Comparator 2/1(Vin), Comparator 3/1(Vin), Comparator 4/1(Vin), Comparator 13/1(Vin), Comparator 12/1(Vin), Comparator 11/1(Vin), Comparator 10/1(Vin), Comparator 9/1(Vin), Comparator 8/1(Vin), Comparator 7/1(Vin), Comparator 6/1(Vin), Comparator 5/1(Vin), Gain1/1
  Vref 14/1 -> Comparator 14/2(Vref)
  Encoder/4(D3) -> D3/1
  Comparator 14/1(b1) -> Encoder/1(b1), Sub DAC/1(b1)
  Comparator 1/1(b2) -> Encoder/2(b2), Sub DAC/2(b2)
  Comparator 2/1(b3) -> Encoder/3(b3), Sub DAC/3(b3)
  Comparator 3/1(b4) -> Encoder/4(b4), Sub DAC/4(b4)
  Comparator 4/1(b5) -> Encoder/5(b5), Sub DAC/5(b5)
  Comparator 5/1(b6) -> Encoder/6(b6), Sub DAC/6(b6)
  Comparator 6/1(b7) -> Encoder/7(b7), Sub DAC/7(b7)
  Comparator 7/1(b8) -> Encoder/8(b8), Sub DAC/8(b8)
  Comparator 8/1(b9) -> Encoder/9(b9), Sub DAC/9(b9)
  Comparator 9/1(b10) -> Encoder/10(b10), Sub DAC/10(b10)
  Comparator 10/1(b11) -> Encoder/11(b11), Sub DAC/11(b11)
  Comparator 11/1(b12) -> Encoder/12(b12), Sub DAC/12(b12)
  Comparator 12/1(b13) -> Encoder/13(b13), Sub DAC/13(b13)
  Comparator 13/1(b14) -> Encoder/14(b14), Sub DAC/14(b14)

== system Sampling_switch_uncertainty/pipeline_13_bit/Adder/Add1 ==
  A : Inport
  B : Inport  Port=2
  Combinatorial Logic1 : CombinatorialLogic  TruthTable=[0 0;1 0 ;1 0;0 1;1 0;0 1;0 1;1 1]
  Constant : Constant  Value=0
  Data Type Conversion : DataTypeConversion  OutDataTypeStr=boolean
  Data Type Conversion1 : DataTypeConversion  OutDataTypeStr=double
  Demux : Demux  Outputs=2
  Mux : Mux  Inputs=3
  Carry : Outport
  Sum : Outport  Port=2
  wires:
  Demux/1 -> Sum/1
  Demux/2 -> Carry/1
  Combinatorial Logic1/1 -> Data Type Conversion1/1
  Mux/1 -> Data Type Conversion/1
  A/1 -> Mux/3
  B/1 -> Mux/2
  Constant/1 -> Mux/1
  Data Type Conversion1/1 -> Demux/1
  Data Type Conversion/1 -> Combinatorial Logic1/1

== system Sampling_switch_uncertainty/pipeline_13_bit/Adder/Add10 ==
  A : Inport
  B : Inport  Port=2
  Combinatorial Logic1 : CombinatorialLogic  TruthTable=[0 0;1 0 ;1 0;0 1;1 0;0 1;0 1;1 1]
  Constant : Constant  Value=0
  Data Type Conversion : DataTypeConversion  OutDataTypeStr=boolean
  Data Type Conversion1 : DataTypeConversion  OutDataTypeStr=double
  Demux : Demux  Outputs=2
  Mux : Mux  Inputs=3
  Carry : Outport
  Sum : Outport  Port=2
  wires:
  Demux/1 -> Sum/1
  Demux/2 -> Carry/1
  Combinatorial Logic1/1 -> Data Type Conversion1/1
  Mux/1 -> Data Type Conversion/1
  A/1 -> Mux/3
  B/1 -> Mux/2
  Constant/1 -> Mux/1
  Data Type Conversion1/1 -> Demux/1
  Data Type Conversion/1 -> Combinatorial Logic1/1

== system Sampling_switch_uncertainty/pipeline_13_bit/Adder/Add11 ==
  A : Inport
  B : Inport  Port=2
  Combinatorial Logic1 : CombinatorialLogic  TruthTable=[0 0;1 0 ;1 0;0 1;1 0;0 1;0 1;1 1]
  Constant : Constant  Value=0
  Data Type Conversion : DataTypeConversion  OutDataTypeStr=boolean
  Data Type Conversion1 : DataTypeConversion  OutDataTypeStr=double
  Demux : Demux  Outputs=2
  Mux : Mux  Inputs=3
  Carry : Outport
  Sum : Outport  Port=2
  wires:
  Demux/1 -> Sum/1
  Demux/2 -> Carry/1
  Combinatorial Logic1/1 -> Data Type Conversion1/1
  Mux/1 -> Data Type Conversion/1
  A/1 -> Mux/3
  B/1 -> Mux/2
  Constant/1 -> Mux/1
  Data Type Conversion1/1 -> Demux/1
  Data Type Conversion/1 -> Combinatorial Logic1/1

== system Sampling_switch_uncertainty/pipeline_13_bit/Adder/Add2 ==
  A : Inport
  B : Inport  Port=2
  C : Inport  Port=3
  Combinatorial Logic1 : CombinatorialLogic  TruthTable=[0 0;1 0 ;1 0;0 1;1 0;0 1;0 1;1 1]
  Data Type Conversion : DataTypeConversion  OutDataTypeStr=boolean
  Data Type Conversion1 : DataTypeConversion  OutDataTypeStr=double
  Demux : Demux  Outputs=2
  Mux : Mux  Inputs=3
  Carry : Outport
  Sum : Outport  Port=2
  wires:
  Demux/1 -> Sum/1
  Demux/2 -> Carry/1
  Combinatorial Logic1/1 -> Data Type Conversion1/1
  Mux/1 -> Data Type Conversion/1
  A/1 -> Mux/3
  B/1 -> Mux/2
  C/1 -> Mux/1
  Data Type Conversion1/1 -> Demux/1
  Data Type Conversion/1 -> Combinatorial Logic1/1

== system Sampling_switch_uncertainty/pipeline_13_bit/Adder/Add3 ==
  A : Inport
  B : Inport  Port=2
  Combinatorial Logic1 : CombinatorialLogic  TruthTable=[0 0;1 0 ;1 0;0 1;1 0;0 1;0 1;1 1]
  Constant : Constant  Value=0
  Data Type Conversion : DataTypeConversion  OutDataTypeStr=boolean
  Data Type Conversion1 : DataTypeConversion  OutDataTypeStr=double
  Demux : Demux  Outputs=2
  Mux : Mux  Inputs=3
  Carry : Outport
  Sum : Outport  Port=2
  wires:
  Demux/1 -> Sum/1
  Demux/2 -> Carry/1
  Combinatorial Logic1/1 -> Data Type Conversion1/1
  Mux/1 -> Data Type Conversion/1
  A/1 -> Mux/3
  B/1 -> Mux/2
  Constant/1 -> Mux/1
  Data Type Conversion1/1 -> Demux/1
  Data Type Conversion/1 -> Combinatorial Logic1/1

== system Sampling_switch_uncertainty/pipeline_13_bit/Adder/Add4 ==
  A : Inport
  B : Inport  Port=2
  C : Inport  Port=3
  Combinatorial Logic1 : CombinatorialLogic  TruthTable=[0 0;1 0 ;1 0;0 1;1 0;0 1;0 1;1 1]
  Data Type Conversion : DataTypeConversion  OutDataTypeStr=boolean
  Data Type Conversion1 : DataTypeConversion  OutDataTypeStr=double
  Demux : Demux  Outputs=2
  Mux : Mux  Inputs=3
  Carry : Outport
  Sum : Outport  Port=2
  wires:
  Demux/1 -> Sum/1
  Demux/2 -> Carry/1
  Combinatorial Logic1/1 -> Data Type Conversion1/1
  Mux/1 -> Data Type Conversion/1
  A/1 -> Mux/3
  B/1 -> Mux/2
  C/1 -> Mux/1
  Data Type Conversion1/1 -> Demux/1
  Data Type Conversion/1 -> Combinatorial Logic1/1

== system Sampling_switch_uncertainty/pipeline_13_bit/Adder/Add5 ==
  A : Inport
  B : Inport  Port=2
  C : Inport  Port=3
  Combinatorial Logic1 : CombinatorialLogic  TruthTable=[0 0;1 0 ;1 0;0 1;1 0;0 1;0 1;1 1]
  Data Type Conversion : DataTypeConversion  OutDataTypeStr=boolean
  Data Type Conversion1 : DataTypeConversion  OutDataTypeStr=double
  Demux : Demux  Outputs=2
  Mux : Mux  Inputs=3
  Carry : Outport
  Sum : Outport  Port=2
  wires:
  Demux/1 -> Sum/1
  Demux/2 -> Carry/1
  Combinatorial Logic1/1 -> Data Type Conversion1/1
  Mux/1 -> Data Type Conversion/1
  A/1 -> Mux/3
  B/1 -> Mux/2
  C/1 -> Mux/1
  Data Type Conversion1/1 -> Demux/1
  Data Type Conversion/1 -> Combinatorial Logic1/1

== system Sampling_switch_uncertainty/pipeline_13_bit/Adder/Add6 ==
  A : Inport
  B : Inport  Port=2
  C : Inport  Port=3
  Combinatorial Logic1 : CombinatorialLogic  TruthTable=[0 0;1 0 ;1 0;0 1;1 0;0 1;0 1;1 1]
  Data Type Conversion : DataTypeConversion  OutDataTypeStr=boolean
  Data Type Conversion1 : DataTypeConversion  OutDataTypeStr=double
  Demux : Demux  Outputs=2
  Mux : Mux  Inputs=3
  Carry : Outport
  Sum : Outport  Port=2
  wires:
  Demux/1 -> Sum/1
  Demux/2 -> Carry/1
  Combinatorial Logic1/1 -> Data Type Conversion1/1
  Mux/1 -> Data Type Conversion/1
  A/1 -> Mux/3
  B/1 -> Mux/2
  C/1 -> Mux/1
  Data Type Conversion1/1 -> Demux/1
  Data Type Conversion/1 -> Combinatorial Logic1/1

== system Sampling_switch_uncertainty/pipeline_13_bit/Adder/Add7 ==
  A : Inport
  B : Inport  Port=2
  C : Inport  Port=3
  Combinatorial Logic1 : CombinatorialLogic  TruthTable=[0 0;1 0 ;1 0;0 1;1 0;0 1;0 1;1 1]
  Data Type Conversion : DataTypeConversion  OutDataTypeStr=boolean
  Data Type Conversion1 : DataTypeConversion  OutDataTypeStr=double
  Demux : Demux  Outputs=2
  Mux : Mux  Inputs=3
  Carry : Outport
  Sum : Outport  Port=2
  wires:
  Demux/1 -> Sum/1
  Demux/2 -> Carry/1
  Combinatorial Logic1/1 -> Data Type Conversion1/1
  Mux/1 -> Data Type Conversion/1
  A/1 -> Mux/3
  B/1 -> Mux/2
  C/1 -> Mux/1
  Data Type Conversion1/1 -> Demux/1
  Data Type Conversion/1 -> Combinatorial Logic1/1

== system Sampling_switch_uncertainty/pipeline_13_bit/Adder/Add8 ==
  A : Inport
  B : Inport  Port=2
  C : Inport  Port=3
  Combinatorial Logic1 : CombinatorialLogic  TruthTable=[0 0;1 0 ;1 0;0 1;1 0;0 1;0 1;1 1]
  Data Type Conversion : DataTypeConversion  OutDataTypeStr=boolean
  Data Type Conversion1 : DataTypeConversion  OutDataTypeStr=double
  Demux : Demux  Outputs=2
  Mux : Mux  Inputs=3
  Carry : Outport
  Sum : Outport  Port=2
  wires:
  Demux/1 -> Sum/1
  Demux/2 -> Carry/1
  Combinatorial Logic1/1 -> Data Type Conversion1/1
  Mux/1 -> Data Type Conversion/1
  A/1 -> Mux/3
  B/1 -> Mux/2
  C/1 -> Mux/1
  Data Type Conversion1/1 -> Demux/1
  Data Type Conversion/1 -> Combinatorial Logic1/1

== system Sampling_switch_uncertainty/pipeline_13_bit/Adder/Add9 ==
  A : Inport
  B : Inport  Port=2
  C : Inport  Port=3
  Combinatorial Logic1 : CombinatorialLogic  TruthTable=[0 0;1 0 ;1 0;0 1;1 0;0 1;0 1;1 1]
  Data Type Conversion : DataTypeConversion  OutDataTypeStr=boolean
  Data Type Conversion1 : DataTypeConversion  OutDataTypeStr=double
  Demux : Demux  Outputs=2
  Mux : Mux  Inputs=3
  Carry : Outport
  Sum : Outport  Port=2
  wires:
  Demux/1 -> Sum/1
  Demux/2 -> Carry/1
  Combinatorial Logic1/1 -> Data Type Conversion1/1
  Mux/1 -> Data Type Conversion/1
  A/1 -> Mux/3
  B/1 -> Mux/2
  C/1 -> Mux/1
  Data Type Conversion1/1 -> Demux/1
  Data Type Conversion/1 -> Combinatorial Logic1/1

== system Sampling_switch_uncertainty/pipeline_13_bit/stage_1p5_bit1/Comparator 1 ==
  Vin : Inport
  Vref : Inport  Port=2
  Output 1 or 0 : Relay  OnSwitchValue=0  OffSwitchValue=0
  Sum : Sum  Inputs=|+-
  Out : Outport
  wires:
  Sum/1 -> Output 1 or 0/1
  Vin/1 -> Sum/1
  Output 1 or 0/1 -> Out/1
  Vref/1 -> Sum/2

== system Sampling_switch_uncertainty/pipeline_13_bit/stage_1p5_bit1/Comparator 2 ==
  Vin : Inport
  Vref : Inport  Port=2
  Output 1 or 0 : Relay  OnSwitchValue=0  OffSwitchValue=0
  Sum : Sum  Inputs=|+-
  Out : Outport
  wires:
  Sum/1 -> Output 1 or 0/1
  Vin/1 -> Sum/1
  Output 1 or 0/1 -> Out/1
  Vref/1 -> Sum/2

== system Sampling_switch_uncertainty/pipeline_13_bit/stage_1p5_bit1/Encoder ==
  b1 : Inport
  b2 : Inport  Port=2
  " " : DataTypeConversion  OutDataTypeStr=double
  NOR : Logic  Operator=NOR  AllPortsSameDT=off  OutDataTypeStr=boolean
  NOT : Logic  Operator=NOT  AllPortsSameDT=off  OutDataTypeStr=boolean
  D0 : Outport
  D1 : Outport  Port=2
  wires:
  b2/1 -> D1/1, NOR/2
  NOR/1 -> " "/1
  " "/1 -> D0/1
  NOT/1 -> NOR/1
  b1/1 -> NOT/1

== system Sampling_switch_uncertainty/pipeline_13_bit/stage_1p5_bit1/Sub DAC ==
  b1 : Inport
  b2 : Inport  Port=2
  NOT : Logic  Operator=NOT  AllPortsSameDT=off  OutDataTypeStr=boolean
  Subtract : Sum  Inputs=-+
  Vdac : Outport
  wires:
  b2/1 -> Subtract/2
  b1/1 -> NOT/1
  Subtract/1 -> Vdac/1
  NOT/1 -> Subtract/1

== system Sampling_switch_uncertainty/pipeline_13_bit/stage_1p5_bit2/Comparator 1 ==
  Vin : Inport
  Vref : Inport  Port=2
  Output 1 or 0 : Relay  OnSwitchValue=0  OffSwitchValue=0
  Sum : Sum  Inputs=|+-
  Out : Outport
  wires:
  Sum/1 -> Output 1 or 0/1
  Vin/1 -> Sum/1
  Output 1 or 0/1 -> Out/1
  Vref/1 -> Sum/2

== system Sampling_switch_uncertainty/pipeline_13_bit/stage_1p5_bit2/Comparator 2 ==
  Vin : Inport
  Vref : Inport  Port=2
  Output 1 or 0 : Relay  OnSwitchValue=0  OffSwitchValue=0
  Sum : Sum  Inputs=|+-
  Out : Outport
  wires:
  Sum/1 -> Output 1 or 0/1
  Vin/1 -> Sum/1
  Output 1 or 0/1 -> Out/1
  Vref/1 -> Sum/2

== system Sampling_switch_uncertainty/pipeline_13_bit/stage_1p5_bit2/Encoder ==
  b1 : Inport
  b2 : Inport  Port=2
  " " : DataTypeConversion  OutDataTypeStr=double
  NOR : Logic  Operator=NOR  AllPortsSameDT=off  OutDataTypeStr=boolean
  NOT : Logic  Operator=NOT  AllPortsSameDT=off  OutDataTypeStr=boolean
  D0 : Outport
  D1 : Outport  Port=2
  wires:
  b2/1 -> D1/1, NOR/2
  NOR/1 -> " "/1
  " "/1 -> D0/1
  NOT/1 -> NOR/1
  b1/1 -> NOT/1

== system Sampling_switch_uncertainty/pipeline_13_bit/stage_1p5_bit2/Sub DAC ==
  b1 : Inport
  b2 : Inport  Port=2
  NOT : Logic  Operator=NOT  AllPortsSameDT=off  OutDataTypeStr=boolean
  Subtract : Sum  Inputs=-+
  Vdac : Outport
  wires:
  b2/1 -> Subtract/2
  b1/1 -> NOT/1
  Subtract/1 -> Vdac/1
  NOT/1 -> Subtract/1

== system Sampling_switch_uncertainty/pipeline_13_bit/stage_1p5_bit3/Comparator 1 ==
  Vin : Inport
  Vref : Inport  Port=2
  Output 1 or 0 : Relay  OnSwitchValue=0  OffSwitchValue=0
  Sum : Sum  Inputs=|+-
  Out : Outport
  wires:
  Sum/1 -> Output 1 or 0/1
  Vin/1 -> Sum/1
  Output 1 or 0/1 -> Out/1
  Vref/1 -> Sum/2

== system Sampling_switch_uncertainty/pipeline_13_bit/stage_1p5_bit3/Comparator 2 ==
  Vin : Inport
  Vref : Inport  Port=2
  Output 1 or 0 : Relay  OnSwitchValue=0  OffSwitchValue=0
  Sum : Sum  Inputs=|+-
  Out : Outport
  wires:
  Sum/1 -> Output 1 or 0/1
  Vin/1 -> Sum/1
  Output 1 or 0/1 -> Out/1
  Vref/1 -> Sum/2

== system Sampling_switch_uncertainty/pipeline_13_bit/stage_1p5_bit3/Encoder ==
  b1 : Inport
  b2 : Inport  Port=2
  " " : DataTypeConversion  OutDataTypeStr=double
  NOR : Logic  Operator=NOR  AllPortsSameDT=off  OutDataTypeStr=boolean
  NOT : Logic  Operator=NOT  AllPortsSameDT=off  OutDataTypeStr=boolean
  D0 : Outport
  D1 : Outport  Port=2
  wires:
  b2/1 -> D1/1, NOR/2
  NOR/1 -> " "/1
  " "/1 -> D0/1
  NOT/1 -> NOR/1
  b1/1 -> NOT/1

== system Sampling_switch_uncertainty/pipeline_13_bit/stage_1p5_bit3/Sub DAC ==
  b1 : Inport
  b2 : Inport  Port=2
  NOT : Logic  Operator=NOT  AllPortsSameDT=off  OutDataTypeStr=boolean
  Subtract : Sum  Inputs=-+
  Vdac : Outport
  wires:
  b2/1 -> Subtract/2
  b1/1 -> NOT/1
  Subtract/1 -> Vdac/1
  NOT/1 -> Subtract/1

== system Sampling_switch_uncertainty/pipeline_13_bit/stage_1p5_bit4/Comparator 1 ==
  Vin : Inport
  Vref : Inport  Port=2
  Output 1 or 0 : Relay  OnSwitchValue=0  OffSwitchValue=0
  Sum : Sum  Inputs=|+-
  Out : Outport
  wires:
  Sum/1 -> Output 1 or 0/1
  Vin/1 -> Sum/1
  Output 1 or 0/1 -> Out/1
  Vref/1 -> Sum/2

== system Sampling_switch_uncertainty/pipeline_13_bit/stage_1p5_bit4/Comparator 2 ==
  Vin : Inport
  Vref : Inport  Port=2
  Output 1 or 0 : Relay  OnSwitchValue=0  OffSwitchValue=0
  Sum : Sum  Inputs=|+-
  Out : Outport
  wires:
  Sum/1 -> Output 1 or 0/1
  Vin/1 -> Sum/1
  Output 1 or 0/1 -> Out/1
  Vref/1 -> Sum/2

== system Sampling_switch_uncertainty/pipeline_13_bit/stage_1p5_bit4/Encoder ==
  b1 : Inport
  b2 : Inport  Port=2
  " " : DataTypeConversion  OutDataTypeStr=double
  NOR : Logic  Operator=NOR  AllPortsSameDT=off  OutDataTypeStr=boolean
  NOT : Logic  Operator=NOT  AllPortsSameDT=off  OutDataTypeStr=boolean
  D0 : Outport
  D1 : Outport  Port=2
  wires:
  b2/1 -> D1/1, NOR/2
  NOR/1 -> " "/1
  " "/1 -> D0/1
  NOT/1 -> NOR/1
  b1/1 -> NOT/1

== system Sampling_switch_uncertainty/pipeline_13_bit/stage_1p5_bit4/Sub DAC ==
  b1 : Inport
  b2 : Inport  Port=2
  NOT : Logic  Operator=NOT  AllPortsSameDT=off  OutDataTypeStr=boolean
  Subtract : Sum  Inputs=-+
  Vdac : Outport
  wires:
  b2/1 -> Subtract/2
  b1/1 -> NOT/1
  Subtract/1 -> Vdac/1
  NOT/1 -> Subtract/1

== system Sampling_switch_uncertainty/pipeline_13_bit/stage_1p5_bit5/Comparator 1 ==
  Vin : Inport
  Vref : Inport  Port=2
  Output 1 or 0 : Relay  OnSwitchValue=0  OffSwitchValue=0
  Sum : Sum  Inputs=|+-
  Out : Outport
  wires:
  Sum/1 -> Output 1 or 0/1
  Vin/1 -> Sum/1
  Output 1 or 0/1 -> Out/1
  Vref/1 -> Sum/2

== system Sampling_switch_uncertainty/pipeline_13_bit/stage_1p5_bit5/Comparator 2 ==
  Vin : Inport
  Vref : Inport  Port=2
  Output 1 or 0 : Relay  OnSwitchValue=0  OffSwitchValue=0
  Sum : Sum  Inputs=|+-
  Out : Outport
  wires:
  Sum/1 -> Output 1 or 0/1
  Vin/1 -> Sum/1
  Output 1 or 0/1 -> Out/1
  Vref/1 -> Sum/2

== system Sampling_switch_uncertainty/pipeline_13_bit/stage_1p5_bit5/Encoder ==
  b1 : Inport
  b2 : Inport  Port=2
  " " : DataTypeConversion  OutDataTypeStr=double
  NOR : Logic  Operator=NOR  AllPortsSameDT=off  OutDataTypeStr=boolean
  NOT : Logic  Operator=NOT  AllPortsSameDT=off  OutDataTypeStr=boolean
  D0 : Outport
  D1 : Outport  Port=2
  wires:
  b2/1 -> D1/1, NOR/2
  NOR/1 -> " "/1
  " "/1 -> D0/1
  NOT/1 -> NOR/1
  b1/1 -> NOT/1

== system Sampling_switch_uncertainty/pipeline_13_bit/stage_1p5_bit5/Sub DAC ==
  b1 : Inport
  b2 : Inport  Port=2
  NOT : Logic  Operator=NOT  AllPortsSameDT=off  OutDataTypeStr=boolean
  Subtract : Sum  Inputs=-+
  Vdac : Outport
  wires:
  b2/1 -> Subtract/2
  b1/1 -> NOT/1
  Subtract/1 -> Vdac/1
  NOT/1 -> Subtract/1

== system Sampling_switch_uncertainty/pipeline_13_bit/stage_1p5_bit6/Comparator 1 ==
  Vin : Inport
  Vref : Inport  Port=2
  Output 1 or 0 : Relay  OnSwitchValue=0  OffSwitchValue=0
  Sum : Sum  Inputs=|+-
  Out : Outport
  wires:
  Sum/1 -> Output 1 or 0/1
  Vin/1 -> Sum/1
  Output 1 or 0/1 -> Out/1
  Vref/1 -> Sum/2

== system Sampling_switch_uncertainty/pipeline_13_bit/stage_1p5_bit6/Comparator 2 ==
  Vin : Inport
  Vref : Inport  Port=2
  Output 1 or 0 : Relay  OnSwitchValue=0  OffSwitchValue=0
  Sum : Sum  Inputs=|+-
  Out : Outport
  wires:
  Sum/1 -> Output 1 or 0/1
  Vin/1 -> Sum/1
  Output 1 or 0/1 -> Out/1
  Vref/1 -> Sum/2

== system Sampling_switch_uncertainty/pipeline_13_bit/stage_1p5_bit6/Encoder ==
  b1 : Inport
  b2 : Inport  Port=2
  " " : DataTypeConversion  OutDataTypeStr=double
  NOR : Logic  Operator=NOR  AllPortsSameDT=off  OutDataTypeStr=boolean
  NOT : Logic  Operator=NOT  AllPortsSameDT=off  OutDataTypeStr=boolean
  D0 : Outport
  D1 : Outport  Port=2
  wires:
  b2/1 -> D1/1, NOR/2
  NOR/1 -> " "/1
  " "/1 -> D0/1
  NOT/1 -> NOR/1
  b1/1 -> NOT/1

== system Sampling_switch_uncertainty/pipeline_13_bit/stage_1p5_bit6/Sub DAC ==
  b1 : Inport
  b2 : Inport  Port=2
  NOT : Logic  Operator=NOT  AllPortsSameDT=off  OutDataTypeStr=boolean
  Subtract : Sum  Inputs=-+
  Vdac : Outport
  wires:
  b2/1 -> Subtract/2
  b1/1 -> NOT/1
  Subtract/1 -> Vdac/1
  NOT/1 -> Subtract/1

== system Sampling_switch_uncertainty/pipeline_13_bit/stage_1p5_bit7/Comparator 1 ==
  Vin : Inport
  Vref : Inport  Port=2
  Output 1 or 0 : Relay  OnSwitchValue=0  OffSwitchValue=0
  Sum : Sum  Inputs=|+-
  Out : Outport
  wires:
  Sum/1 -> Output 1 or 0/1
  Vin/1 -> Sum/1
  Output 1 or 0/1 -> Out/1
  Vref/1 -> Sum/2

== system Sampling_switch_uncertainty/pipeline_13_bit/stage_1p5_bit7/Comparator 2 ==
  Vin : Inport
  Vref : Inport  Port=2
  Output 1 or 0 : Relay  OnSwitchValue=0  OffSwitchValue=0
  Sum : Sum  Inputs=|+-
  Out : Outport
  wires:
  Sum/1 -> Output 1 or 0/1
  Vin/1 -> Sum/1
  Output 1 or 0/1 -> Out/1
  Vref/1 -> Sum/2

== system Sampling_switch_uncertainty/pipeline_13_bit/stage_1p5_bit7/Encoder ==
  b1 : Inport
  b2 : Inport  Port=2
  " " : DataTypeConversion  OutDataTypeStr=double
  NOR : Logic  Operator=NOR  AllPortsSameDT=off  OutDataTypeStr=boolean
  NOT : Logic  Operator=NOT  AllPortsSameDT=off  OutDataTypeStr=boolean
  D0 : Outport
  D1 : Outport  Port=2
  wires:
  b2/1 -> D1/1, NOR/2
  NOR/1 -> " "/1
  " "/1 -> D0/1
  NOT/1 -> NOR/1
  b1/1 -> NOT/1

== system Sampling_switch_uncertainty/pipeline_13_bit/stage_1p5_bit7/Sub DAC ==
  b1 : Inport
  b2 : Inport  Port=2
  NOT : Logic  Operator=NOT  AllPortsSameDT=off  OutDataTypeStr=boolean
  Subtract : Sum  Inputs=-+
  Vdac : Outport
  wires:
  b2/1 -> Subtract/2
  b1/1 -> NOT/1
  Subtract/1 -> Vdac/1
  NOT/1 -> Subtract/1

== system Sampling_switch_uncertainty/pipeline_13_bit/stage_3_bit_flash/Comparator 1 ==
  Vin : Inport
  Vref : Inport  Port=2
  Output 1 or 0 : Relay  OnSwitchValue=0  OffSwitchValue=0
  Sum : Sum  Inputs=|+-
  Out : Outport
  wires:
  Sum/1 -> Output 1 or 0/1
  Vin/1 -> Sum/1
  Output 1 or 0/1 -> Out/1
  Vref/1 -> Sum/2

== system Sampling_switch_uncertainty/pipeline_13_bit/stage_3_bit_flash/Comparator 2 ==
  Vin : Inport
  Vref : Inport  Port=2
  Output 1 or 0 : Relay  OnSwitchValue=0  OffSwitchValue=0
  Sum : Sum  Inputs=|+-
  Out : Outport
  wires:
  Sum/1 -> Output 1 or 0/1
  Vin/1 -> Sum/1
  Output 1 or 0/1 -> Out/1
  Vref/1 -> Sum/2

== system Sampling_switch_uncertainty/pipeline_13_bit/stage_3_bit_flash/Comparator 3 ==
  Vin : Inport
  Vref : Inport  Port=2
  Output 1 or 0 : Relay  OnSwitchValue=0  OffSwitchValue=0
  Sum : Sum  Inputs=|+-
  Out : Outport
  wires:
  Sum/1 -> Output 1 or 0/1
  Vin/1 -> Sum/1
  Output 1 or 0/1 -> Out/1
  Vref/1 -> Sum/2

== system Sampling_switch_uncertainty/pipeline_13_bit/stage_3_bit_flash/Comparator 4 ==
  Vin : Inport
  Vref : Inport  Port=2
  Output 1 or 0 : Relay  OnSwitchValue=0  OffSwitchValue=0
  Sum : Sum  Inputs=|+-
  Out : Outport
  wires:
  Sum/1 -> Output 1 or 0/1
  Vin/1 -> Sum/1
  Output 1 or 0/1 -> Out/1
  Vref/1 -> Sum/2

== system Sampling_switch_uncertainty/pipeline_13_bit/stage_3_bit_flash/Comparator 5 ==
  Vin : Inport
  Vref : Inport  Port=2
  Output 1 or 0 : Relay  OnSwitchValue=0  OffSwitchValue=0
  Sum : Sum  Inputs=|+-
  Out : Outport
  wires:
  Sum/1 -> Output 1 or 0/1
  Vin/1 -> Sum/1
  Output 1 or 0/1 -> Out/1
  Vref/1 -> Sum/2

== system Sampling_switch_uncertainty/pipeline_13_bit/stage_3_bit_flash/Comparator 6 ==
  Vin : Inport
  Vref : Inport  Port=2
  Output 1 or 0 : Relay  OnSwitchValue=0  OffSwitchValue=0
  Sum : Sum  Inputs=|+-
  Out : Outport
  wires:
  Sum/1 -> Output 1 or 0/1
  Vin/1 -> Sum/1
  Output 1 or 0/1 -> Out/1
  Vref/1 -> Sum/2

== system Sampling_switch_uncertainty/pipeline_13_bit/stage_3_bit_flash/Comparator 7 ==
  Vin : Inport
  Vref : Inport  Port=2
  Output 1 or 0 : Relay  OnSwitchValue=0  OffSwitchValue=0
  Sum : Sum  Inputs=|+-
  Out : Outport
  wires:
  Sum/1 -> Output 1 or 0/1
  Vin/1 -> Sum/1
  Output 1 or 0/1 -> Out/1
  Vref/1 -> Sum/2

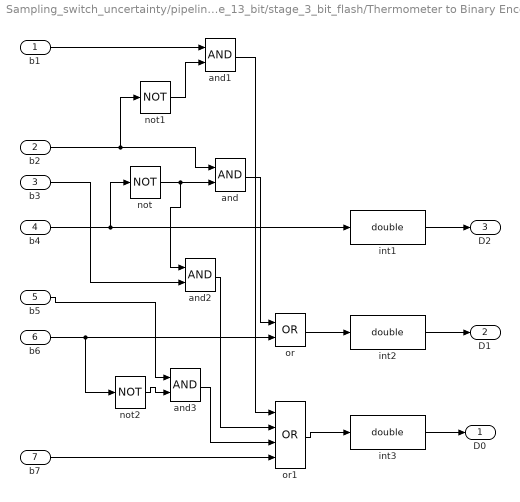
== system Sampling_switch_uncertainty/pipeline_13_bit/stage_3_bit_flash/Thermometer to Binary Encoder ==
  b1 : Inport
  b2 : Inport  Port=2
  b3 : Inport  Port=3
  b4 : Inport  Port=4
  b5 : Inport  Port=5
  b6 : Inport  Port=6
  b7 : Inport  Port=7
  and{,1..3} (4 alike) : Logic  AllPortsSameDT=off  OutDataTypeStr=boolean
  int1 : DataTypeConversion  OutDataTypeStr=double
  int2 : DataTypeConversion  OutDataTypeStr=double
  int3 : DataTypeConversion  OutDataTypeStr=double
  not : Logic  Operator=NOT  AllPortsSameDT=off  OutDataTypeStr=boolean
  not1 : Logic  Operator=NOT  AllPortsSameDT=off  OutDataTypeStr=boolean
  not2 : Logic  Operator=NOT  AllPortsSameDT=off  OutDataTypeStr=boolean
  or : Logic  Operator=OR  AllPortsSameDT=off  OutDataTypeStr=boolean
  or1 : Logic  Operator=OR  Inputs=4  AllPortsSameDT=off  OutDataTypeStr=boolean
  D0 : Outport
  D1 : Outport  Port=2
  D2 : Outport  Port=3
  wires:
  b4/1 -> not/1, int1/1
  not/1 -> and/2, and2/1
  b2/1 -> and/1, not1/1
  b6/1 -> or/2, not2/1
  and/1 -> or/1
  or/1 -> int2/1
  or1/1 -> int3/1
  b1/1 -> and1/1
  not1/1 -> and1/2
  and1/1 -> or1/1
  b3/1 -> and2/2
  and2/1 -> or1/2
  b7/1 -> or1/4
  not2/1 -> and3/2
  b5/1 -> and3/1
  int2/1 -> D1/1
  int3/1 -> D0/1
  and3/1 -> or1/3
  int1/1 -> D2/1

== system Sampling_switch_uncertainty/pipeline_13_bit/stage_3p5_bit/Comparator 1 ==
  Vin : Inport
  Vref : Inport  Port=2
  Output 1 or 0 : Relay  OnSwitchValue=0  OffSwitchValue=0
  Sum : Sum  Inputs=|+-
  b2 : Outport
  wires:
  Sum/1 -> Output 1 or 0/1
  Vin/1 -> Sum/1
  Output 1 or 0/1 -> b2/1
  Vref/1 -> Sum/2

== system Sampling_switch_uncertainty/pipeline_13_bit/stage_3p5_bit/Comparator 10 ==
  Vin : Inport
  Vref : Inport  Port=2
  Output 1 or 0 : Relay  OnSwitchValue=0  OffSwitchValue=0
  Sum : Sum  Inputs=|+-
  b11 : Outport
  wires:
  Sum/1 -> Output 1 or 0/1
  Vin/1 -> Sum/1
  Output 1 or 0/1 -> b11/1
  Vref/1 -> Sum/2

== system Sampling_switch_uncertainty/pipeline_13_bit/stage_3p5_bit/Comparator 11 ==
  Vin : Inport
  Vref : Inport  Port=2
  Output 1 or 0 : Relay  OnSwitchValue=0  OffSwitchValue=0
  Sum : Sum  Inputs=|+-
  b12 : Outport
  wires:
  Sum/1 -> Output 1 or 0/1
  Vin/1 -> Sum/1
  Output 1 or 0/1 -> b12/1
  Vref/1 -> Sum/2

== system Sampling_switch_uncertainty/pipeline_13_bit/stage_3p5_bit/Comparator 12 ==
  Vin : Inport
  Vref : Inport  Port=2
  Output 1 or 0 : Relay  OnSwitchValue=0  OffSwitchValue=0
  Sum : Sum  Inputs=|+-
  b13 : Outport
  wires:
  Sum/1 -> Output 1 or 0/1
  Vin/1 -> Sum/1
  Output 1 or 0/1 -> b13/1
  Vref/1 -> Sum/2

== system Sampling_switch_uncertainty/pipeline_13_bit/stage_3p5_bit/Comparator 13 ==
  Vin : Inport
  Vref : Inport  Port=2
  Output 1 or 0 : Relay  OnSwitchValue=0  OffSwitchValue=0
  Sum : Sum  Inputs=|+-
  b14 : Outport
  wires:
  Sum/1 -> Output 1 or 0/1
  Vin/1 -> Sum/1
  Output 1 or 0/1 -> b14/1
  Vref/1 -> Sum/2

== system Sampling_switch_uncertainty/pipeline_13_bit/stage_3p5_bit/Comparator 14 ==
  Vin : Inport
  Vref : Inport  Port=2
  Output 1 or 0 : Relay  OnSwitchValue=0  OffSwitchValue=0
  Sum : Sum  Inputs=|+-
  b1 : Outport
  wires:
  Sum/1 -> Output 1 or 0/1
  Vin/1 -> Sum/1
  Output 1 or 0/1 -> b1/1
  Vref/1 -> Sum/2

== system Sampling_switch_uncertainty/pipeline_13_bit/stage_3p5_bit/Comparator 2 ==
  Vin : Inport
  Vref : Inport  Port=2
  Output 1 or 0 : Relay  OnSwitchValue=0  OffSwitchValue=0
  Sum : Sum  Inputs=|+-
  b3 : Outport
  wires:
  Sum/1 -> Output 1 or 0/1
  Vin/1 -> Sum/1
  Output 1 or 0/1 -> b3/1
  Vref/1 -> Sum/2

== system Sampling_switch_uncertainty/pipeline_13_bit/stage_3p5_bit/Comparator 3 ==
  Vin : Inport
  Vref : Inport  Port=2
  Output 1 or 0 : Relay  OnSwitchValue=0  OffSwitchValue=0
  Sum : Sum  Inputs=|+-
  b4 : Outport
  wires:
  Sum/1 -> Output 1 or 0/1
  Vin/1 -> Sum/1
  Output 1 or 0/1 -> b4/1
  Vref/1 -> Sum/2

== system Sampling_switch_uncertainty/pipeline_13_bit/stage_3p5_bit/Comparator 4 ==
  Vin : Inport
  Vref : Inport  Port=2
  Output 1 or 0 : Relay  OnSwitchValue=0  OffSwitchValue=0
  Sum : Sum  Inputs=|+-
  b5 : Outport
  wires:
  Sum/1 -> Output 1 or 0/1
  Vin/1 -> Sum/1
  Output 1 or 0/1 -> b5/1
  Vref/1 -> Sum/2

== system Sampling_switch_uncertainty/pipeline_13_bit/stage_3p5_bit/Comparator 5 ==
  Vin : Inport
  Vref : Inport  Port=2
  Output 1 or 0 : Relay  OnSwitchValue=0  OffSwitchValue=0
  Sum : Sum  Inputs=|+-
  b6 : Outport
  wires:
  Sum/1 -> Output 1 or 0/1
  Vin/1 -> Sum/1
  Output 1 or 0/1 -> b6/1
  Vref/1 -> Sum/2

== system Sampling_switch_uncertainty/pipeline_13_bit/stage_3p5_bit/Comparator 6 ==
  Vin : Inport
  Vref : Inport  Port=2
  Output 1 or 0 : Relay  OnSwitchValue=0  OffSwitchValue=0
  Sum : Sum  Inputs=|+-
  b7 : Outport
  wires:
  Sum/1 -> Output 1 or 0/1
  Vin/1 -> Sum/1
  Output 1 or 0/1 -> b7/1
  Vref/1 -> Sum/2

== system Sampling_switch_uncertainty/pipeline_13_bit/stage_3p5_bit/Comparator 7 ==
  Vin : Inport
  Vref : Inport  Port=2
  Output 1 or 0 : Relay  OnSwitchValue=0  OffSwitchValue=0
  Sum : Sum  Inputs=|+-
  b8 : Outport
  wires:
  Sum/1 -> Output 1 or 0/1
  Vin/1 -> Sum/1
  Output 1 or 0/1 -> b8/1
  Vref/1 -> Sum/2

== system Sampling_switch_uncertainty/pipeline_13_bit/stage_3p5_bit/Comparator 8 ==
  Vin : Inport
  Vref : Inport  Port=2
  Output 1 or 0 : Relay  OnSwitchValue=0  OffSwitchValue=0
  Sum : Sum  Inputs=|+-
  b9 : Outport
  wires:
  Sum/1 -> Output 1 or 0/1
  Vin/1 -> Sum/1
  Output 1 or 0/1 -> b9/1
  Vref/1 -> Sum/2

== system Sampling_switch_uncertainty/pipeline_13_bit/stage_3p5_bit/Comparator 9 ==
  Vin : Inport
  Vref : Inport  Port=2
  Output 1 or 0 : Relay  OnSwitchValue=0  OffSwitchValue=0
  Sum : Sum  Inputs=|+-
  b10 : Outport
  wires:
  Sum/1 -> Output 1 or 0/1
  Vin/1 -> Sum/1
  Output 1 or 0/1 -> b10/1
  Vref/1 -> Sum/2
